simulink model "pendulum"  (R2024a)
settings: Solver=VariableStepAuto  StartTime=0.0  StopTime=10  FixedStep=0.01  MaxStep=1e-2
model workspace (MAT data in the model file):
  L = 0.2
  M = 0.054
  b = 0.01
  g = 9.81
undefined symbols (not defined in the file): X, Y, Z
libraries: sm_lib x6, nesl_utility x4
settings Model: Creator=zrway  LastModifiedBy=zrway

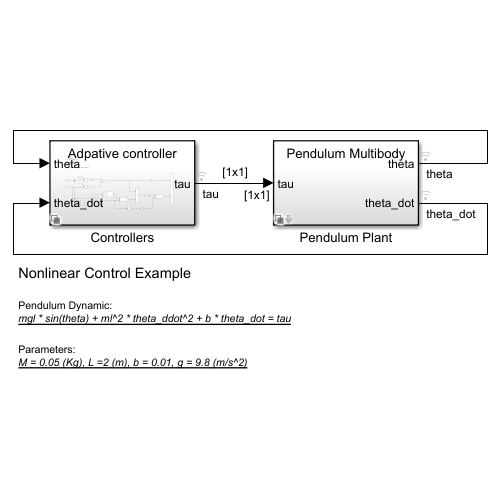
[thumbnail: Simulink's stored preview of the top-level diagram]
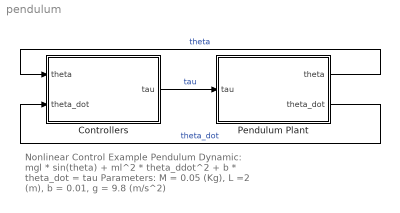
== system pendulum ==
  note: Nonlinear Control Example
      |
      | Pendulum Dynamic:
      | mgl * sin(theta) + ml^2 * theta_ddot^2 + b * theta_dot = tau
      |
      | Parameters:
      | M = 0.05 (Kg), L =2 (m), b = 0.01, g = 9.8 (m/s^2)
  Controllers : Subsystem  Variant=on  VariantControlMode=label  VariantControl=PFL controller  LabelModeActiveChoice=Adpative controller
  Pendulum Plant : Subsystem  Variant=on  VariantControlMode=label  VariantControl=Pendulum with Friction  LabelModeActiveChoice=Pendulum Multibody
  wires:
  Controllers/1(tau) -> Pendulum Plant/1(tau)  "tau"
  Pendulum Plant/1(theta) -> Controllers/1(theta)  "theta"
  Pendulum Plant/2(theta_dot) -> Controllers/2(theta_dot)  "theta_dot"

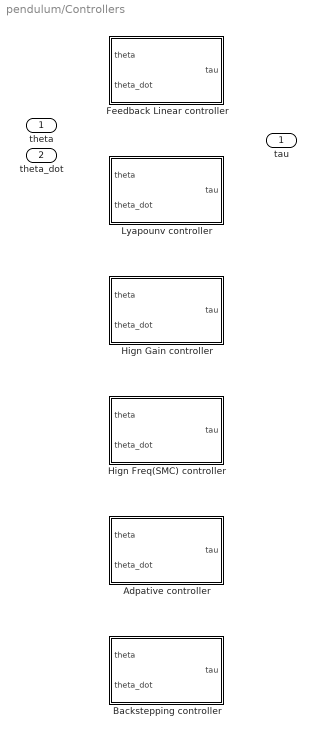
== system pendulum/Controllers ==
  theta : Inport
  theta_dot : Inport  Port=2
  Adpative controller : Subsystem  VariantControl=Adpative controller
  Backstepping controller : Subsystem  Variant=on  VariantControlMode=label  VariantControl=Backstepping controller  LabelModeActiveChoice=Backstepping controller2
  Feedback Linear controller : Subsystem  VariantControl=Feedback Linear controller
  Hign Freq(SMC) controller : Subsystem  VariantControl=Hign Freq(SMC) controller
  Hign Gain controller : Subsystem  VariantControl=Hign Gain controller
  Lyapounv controller : Subsystem  VariantControl=Lyapounv controller
  tau : Outport

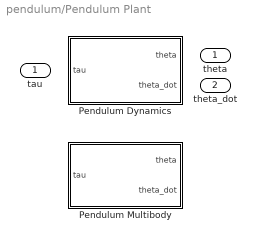
== system pendulum/Pendulum Plant ==
  tau : Inport
  Pendulum Dynamics : Subsystem  VariantControl=Pendulum Dynamics
  Pendulum Multibody : Subsystem  VariantControl=Pendulum Multibody  mask(Pendulum){L=L, W=0.01, H=0.01, m=M, rgb=[0.25 0.40 0.70], theta_init=0.4, b=b}
      mask prompts: L "Length (m)"; W "Width (m)"; H "Thickness (m)"; m "Mass (kg)"; rgb "Color [R G B]"; theta_init "Initial q (rad)"; b "Damping ratio (N*m*s/rad)"
      mask help: Pendulum simscape multibody block.
  theta : Outport
  theta_dot : Outport  Port=2

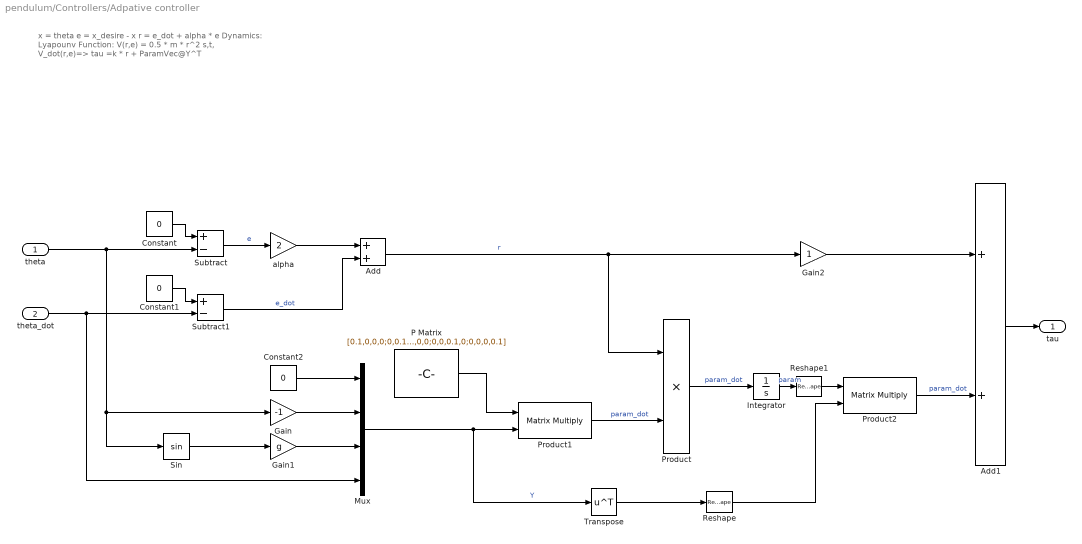
== system pendulum/Controllers/Adpative controller ==
  note: x = theta
      | e = x_desire - x
      | r = e_dot + alpha * e
      |
      | Dynamics:
      | Lyapounv Function:
      | V(r,e) = 0.5 * m * r^2
      |
      | s,t, V_dot(r,e)=> tau =k * r + ParamVec@Y^T
  theta : Inport
  theta_dot : Inport  Port=2
  Add : Sum
  Add1 : Sum
  Constant : Constant  Value=0
  Constant1 : Constant  Value=0
  Constant2 : Constant  Value=0
  Gain : Gain  Gain=-1
  Gain1 : Gain  Gain=g
  Gain2 : Gain
  Integrator : Integrator  InitialCondition=[1,0.2,1,0.1]
  Mux : Mux
  P Matrix : Constant  Value=[0.1,0,0,0;0,0.1,0,0;0,0,0.1,0;0,0,0,0.1]
  Product : Product
  Product1 : Product  Multiplication=Matrix(*)
  Product2 : Product  Multiplication=Matrix(*)
  Reshape : Reshape  OutputDimensionality=Column vector (2-D)
  Reshape1 : Reshape  OutputDimensionality=Row vector (2-D)
  Sin : Trigonometry
  Subtract : Sum  Inputs=+-
  Subtract1 : Sum  Inputs=+-
  Transpose : Math  Operator=transpose
  alpha : Gain  Gain=2
  tau : Outport
  wires:
  Subtract/1 -> alpha/1  "e"
  theta_dot/1 -> Mux/4, Subtract1/2
  theta/1 -> Sin/1, Gain/1, Subtract/2
  Add/1 -> Gain2/1, Product/1  "r"
  alpha/1 -> Add/1
  Subtract1/1 -> Add/2  "e_dot"
  Constant/1 -> Subtract/1
  Constant1/1 -> Subtract1/1
  Product/1 -> Integrator/1  "param_dot"
  Constant2/1 -> Mux/1
  Gain/1 -> Mux/2
  Gain1/1 -> Mux/3
  Sin/1 -> Gain1/1
  Mux/1 -> Transpose/1, Product1/2  "Y"
  P Matrix/1 -> Product1/1
  Product1/1 -> Product/2  "param_dot"
  Integrator/1 -> Reshape1/1  "param"
  Transpose/1 -> Reshape/1
  Product2/1 -> Add1/2  "param_dot"
  Gain2/1 -> Add1/1
  Add1/1 -> tau/1
  Reshape/1 -> Product2/2
  Reshape1/1 -> Product2/1

== system pendulum/Controllers/Backstepping controller ==
  theta : Inport
  theta_dot : Inport  Port=2
  Backstepping controller1 : Subsystem  VariantControl=Backstepping controller
  Backstepping controller2 : Subsystem  VariantControl=Backstepping controller2
  tau : Outport

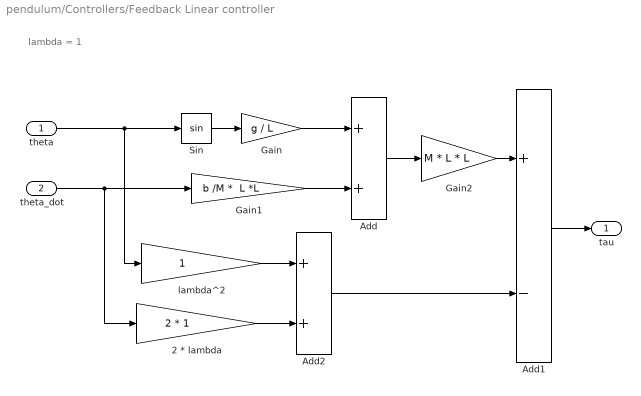
== system pendulum/Controllers/Feedback Linear controller ==
  note: lambda = 1
  theta : Inport
  theta_dot : Inport  Port=2
  2 * lambda : Gain  Gain=2 * 1
  Add : Sum
  Add1 : Sum  Inputs=+-
  Add2 : Sum
  Gain : Gain  Gain=g / L
  Gain1 : Gain  Gain="b /M *  L *L"
  Gain2 : Gain  Gain=M * L * L
  Sin : Trigonometry
  lambda^2 : Gain
  tau : Outport
  wires:
  theta/1 -> Sin/1, lambda^2/1
  Sin/1 -> Gain/1
  theta_dot/1 -> 2 * lambda/1, Gain1/1
  Gain/1 -> Add/1
  Gain1/1 -> Add/2
  Add/1 -> Gain2/1
  Gain2/1 -> Add1/1
  Add1/1 -> tau/1
  Add2/1 -> Add1/2
  2 * lambda/1 -> Add2/2
  lambda^2/1 -> Add2/1

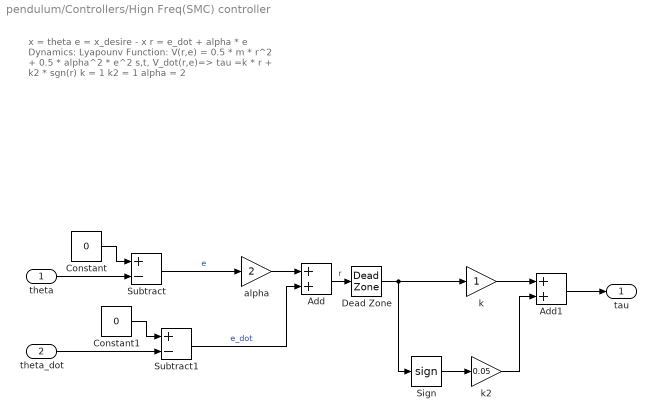
== system pendulum/Controllers/Hign Freq(SMC) controller ==
  note: x = theta
      | e = x_desire - x
      | r = e_dot + alpha * e
      |
      | Dynamics:
      | Lyapounv Function:
      | V(r,e) = 0.5 * m * r^2 + 0.5 * alpha^2 * e^2
      |
      | s,t, V_dot(r,e)=> tau =k * r + k2 * sgn(r)
      |
      | k = 1
      | k2 = 1
      | alpha = 2
  theta : Inport
  theta_dot : Inport  Port=2
  Add : Sum
  Add1 : Sum
  Constant : Constant  Value=0
  Constant1 : Constant  Value=0
  Dead Zone : DeadZone  LowerValue=-0.01  UpperValue=0.01
  Sign : Signum
  Subtract : Sum  Inputs=+-
  Subtract1 : Sum  Inputs=+-
  alpha : Gain  Gain=2
  k : Gain
  k2 : Gain  Gain=0.05
  tau : Outport
  wires:
  Constant/1 -> Subtract/1
  theta/1 -> Subtract/2
  Subtract1/1 -> Add/2  "e_dot"
  alpha/1 -> Add/1
  Subtract/1 -> alpha/1  "e"
  Add/1 -> Dead Zone/1  "r"
  theta_dot/1 -> Subtract1/2
  Constant1/1 -> Subtract1/1
  k/1 -> Add1/1
  Sign/1 -> k2/1
  k2/1 -> Add1/2
  Add1/1 -> tau/1
  Dead Zone/1 -> Sign/1, k/1

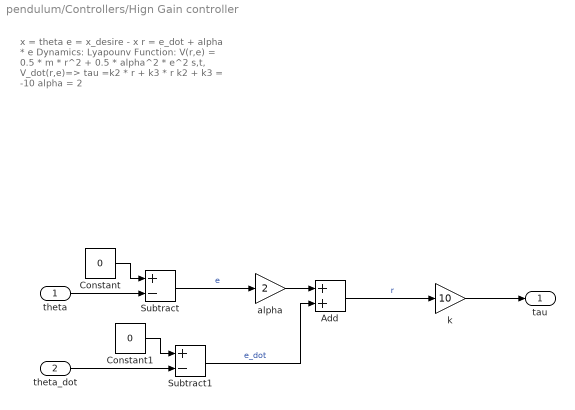
== system pendulum/Controllers/Hign Gain controller ==
  note: x = theta
      | e = x_desire - x
      | r = e_dot + alpha * e
      |
      | Dynamics:
      | Lyapounv Function:
      | V(r,e) = 0.5 * m * r^2 + 0.5 * alpha^2 * e^2
      |
      | s,t, V_dot(r,e)=> tau =k2 * r + k3 * r
      |
      | k2 + k3 = -10
      | alpha = 2
  theta : Inport
  theta_dot : Inport  Port=2
  Add : Sum
  Constant : Constant  Value=0
  Constant1 : Constant  Value=0
  Subtract : Sum  Inputs=+-
  Subtract1 : Sum  Inputs=+-
  alpha : Gain  Gain=2
  k : Gain  Gain=10
  tau : Outport
  wires:
  k/1 -> tau/1
  alpha/1 -> Add/1
  Add/1 -> k/1  "r"
  Constant/1 -> Subtract/1
  theta/1 -> Subtract/2
  Subtract/1 -> alpha/1  "e"
  Constant1/1 -> Subtract1/1
  theta_dot/1 -> Subtract1/2
  Subtract1/1 -> Add/2  "e_dot"

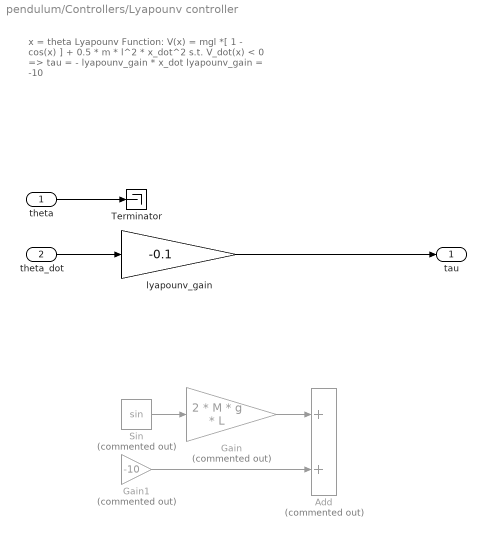
== system pendulum/Controllers/Lyapounv controller ==
  note: x = theta
      |
      | Lyapounv Function:
      | V(x) = mgl *[ 1 - cos(x) ] + 0.5 * m * l^2 * x_dot^2
      | s.t. V_dot(x) < 0
      | => tau = - lyapounv_gain * x_dot
      |
      | lyapounv_gain = -10
  theta : Inport
  theta_dot : Inport  Port=2
  Add : Sum  Commented=on
  Gain : Gain  Commented=on  Gain=2 * M * g * L
  Gain1 : Gain  Commented=on  Gain=-10
  Sin : Trigonometry  Commented=on
  Terminator : Terminator
  lyapounv_gain : Gain  Gain=-0.1
  tau : Outport
  wires:
  Sin/1 -> Gain/1
  Gain1/1 -> Add/2
  Gain/1 -> Add/1
  theta_dot/1 -> lyapounv_gain/1
  theta/1 -> Terminator/1
  lyapounv_gain/1 -> tau/1

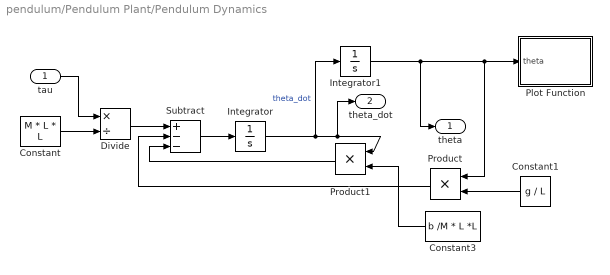
== system pendulum/Pendulum Plant/Pendulum Dynamics ==
  tau : Inport
  Constant : Constant  Value=M * L * L
  Constant1 : Constant  Value=g / L
  Constant3 : Constant  Value="b /M *  L *L"
  Divide : Product  Inputs=*/
  Integrator : Integrator
  Integrator1 : Integrator  InitialCondition=0.4  WrapState=on
  Plot Function : MATLAB Function  TreatAsAtomicUnit=on
  Product : Product
  Product1 : Product
  Subtract : Sum  Inputs=+--
  theta : Outport
  theta_dot : Outport  Port=2
  wires:
  Constant3/1 -> Product1/2
  Constant/1 -> Divide/2
  Constant1/1 -> Product/2
  tau/1 -> Divide/1
  Integrator/1 -> Product1/1, theta_dot/1, Integrator1/1  "theta_dot"
  Divide/1 -> Subtract/1
  Subtract/1 -> Integrator/1
  Product/1 -> Subtract/2
  Product1/1 -> Subtract/3
  Integrator1/1 -> Plot Function/1(theta), Product/1, theta/1

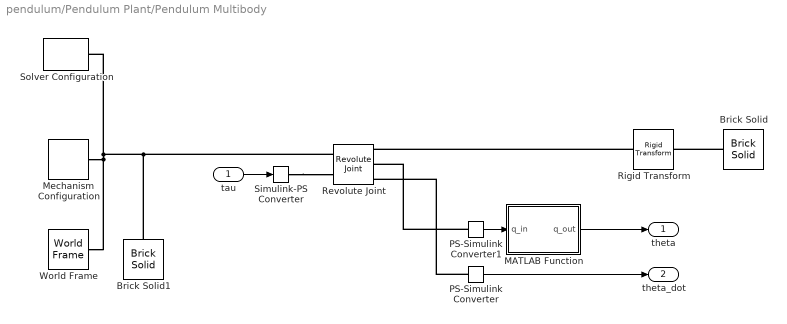
== system pendulum/Pendulum Plant/Pendulum Multibody ==
  tau : Inport
  Brick Solid : sm_lib/Body Elements/Brick Solid  BrickDimensions=[L H W]  BrickDimensionsUnits=m  ExportEntireGeometry=off  InertiaType=CalculateFromGeometry  BasedOnType=Mass  Density=rho  DensityUnits=kg/m^3  Mass=m  MassUnits=kg  CenterOfMass=[0 0 0]  CenterOfMassUnits=m  MomentsOfInertia=[1 1 1]  MomentsOfInertiaUnits=kg*m^2  ProductsOfInertia=[0 0 0]  ProductsOfInertiaUnits=kg*m^2  GraphicType=FromGeometry  MarkerShape=Sphere  MarkerSize=10  GraphicVisPropType=SimpleVisualProperties  GraphicDiffuseColor=rgb  GraphicOpacity=1  GraphicSpecularColor=[0.5 0.5 0.5 1.0]  GraphicAmbientColor=[0.15 0.15 0.15 1.0]  GraphicEmissiveColor=[0.0 0.0 0.0 1.0]  GraphicShininess=75  DoExposeReferenceFrame=on  SerializedFrames=<Frames/>
  Brick Solid1 : sm_lib/Body Elements/Brick Solid  BrickDimensions=[0.04 0.04 0.04]  BrickDimensionsUnits=m  ExportEntireGeometry=off  InertiaType=CalculateFromGeometry  BasedOnType=Density  Density=1000  DensityUnits=kg/m^3  Mass=1  MassUnits=kg  CenterOfMass=[0 0 0]  CenterOfMassUnits=m  MomentsOfInertia=[1 1 1]  MomentsOfInertiaUnits=kg*m^2  ProductsOfInertia=[0 0 0]  ProductsOfInertiaUnits=kg*m^2  GraphicType=FromGeometry  MarkerShape=Sphere  MarkerSize=10  GraphicVisPropType=SimpleVisualProperties  GraphicDiffuseColor=[0.80 0.45 0]  GraphicOpacity=1  GraphicSpecularColor=[0.5 0.5 0.5 1.0]  GraphicAmbientColor=[0.15 0.15 0.15 1.0]  GraphicEmissiveColor=[0.0 0.0 0.0 1.0]  GraphicShininess=75  DoExposeReferenceFrame=on  SerializedFrames=<Frames/>
  MATLAB Function : MATLAB Function  TreatAsAtomicUnit=on
  Mechanism Configuration : sm_lib/Utilities/Mechanism Configuration  UniformGravity=Constant  GravityVector=[0 -9.80665 0]  GravityVectorUnits=m/s^2  LinearizationDelta=0.001  JointModeTransitionNonlinearIterations=2
  PS-Simulink Converter : nesl_utility/PS-Simulink Converter  PhysicalDomain=network_engine_domain  SubClassName=ps_output  LeftPortType=input  RightPortType=output  PseudoPeriodic=off  Frequencies=[]  VectorFormat=1-D array  Unit=rad/s  AffineConversion=off
  PS-Simulink Converter1 : nesl_utility/PS-Simulink Converter  PhysicalDomain=network_engine_domain  SubClassName=ps_output  LeftPortType=input  RightPortType=output  PseudoPeriodic=off  Frequencies=[]  VectorFormat=inherit  Unit=rad  AffineConversion=off
  Revolute Joint : sm_lib/Joints/Revolute Joint  JointMode=Normal  CompositeWrenchDir=FollowerOnBase  CompositeWrenchFrame=BaseFrame  SenseConstraintForce=off  SenseConstraintTorque=off  SenseTotalForce=off  SenseTotalTorque=off  PositionTargetSpecify=on  PositionTargetPriority=High  PositionTargetValue=-pi / 2 + theta_init  PositionTargetValueUnits=rad  VelocityTargetSpecify=on  VelocityTargetPriority=Low  VelocityTargetValue=0.0001  VelocityTargetValueUnits=rad/s  EquilibriumPosition=pi / 2  EquilibriumPositionUnits=rad  SpringStiffness=0  SpringStiffnessUnits=N*m/deg  DampingCoefficient=b  DampingCoefficientUnits=N*m*s/rad  LowerLimitSpecify=off  LowerLimitBound=-90  LowerLimitBoundUnits=deg  LowerLimitStiffness=1e4  LowerLimitStiffnessUnits=N*m/deg  LowerLimitDamping=10  LowerLimitDampingUnits=N*m/(deg/s)  LowerLimitTransitionRegionWidth=0.1  LowerLimitTransitionRegionWidthUnits=deg  UpperLimitSpecify=off  UpperLimitBound=90  UpperLimitBoundUnits=deg  UpperLimitStiffness=1e4  UpperLimitStiffnessUnits=N*m/deg  UpperLimitDamping=10  UpperLimitDampingUnits=N*m/(deg/s)  UpperLimitTransitionRegionWidth=0.1  UpperLimitTransitionRegionWidthUnits=deg  TorqueActuationMode=InputTorque  MotionActuationMode=ComputedMotion  SensePosition=on  SenseVelocity=on  SenseAcceleration=off  SenseTorqueForce=off  SenseLowerLimitTorqueForce=off  SenseUpperLimitTorqueForce=off
  Rigid Transform : sm_lib/Frames and Transforms/Rigid Transform  RotationMethod=None  FollAlignAxisA=+X  BaseAlignAxisA=+Y  FollAlignAxisB=+Y  BaseAlignAxisB=+Z  RotationStandardAxis=+Z  RotationAngle=0  RotationAngleUnits=deg  RotationArbitraryAxis=[0 0 1]  RotationSequenceAxes=FollowerAxes  RotationSequence=XYX  RotationSequenceAngles=[0 0 0]  RotationSequenceAnglesUnits=deg  RotationMatrix=[1 0 0;0 1 0;0 0 1]  Quaternion=[1 0 0 0]  TranslationMethod=StandardAxis  TranslationCartesianOffset=[0 0 0]  TranslationCartesianOffsetUnits=m  TranslationStandardAxis=-X  TranslationStandardOffset=L / 2  TranslationStandardOffsetUnits=m  TranslationROffset=0  TranslationROffsetUnits=m  TranslationThetaOffset=0  TranslationThetaOffsetUnits=deg  TranslationZOffset=0  TranslationZOffsetUnits=m
  Simulink-PS Converter : nesl_utility/Simulink-PS Converter  PhysicalDomain=network_engine_domain  SubClassName=ps_input  LeftPortType=input  RightPortType=output  PseudoPeriodic=off  Frequencies=[]  NoiseDistribution=none  NoiseParameters=[]  Unit=N*m  AffineConversion=off  FilteringAndDerivatives=provide  SimscapeFilterOrder=1  InputFilterTimeConstant=0.001  UdotUserProvided=0
  Solver Configuration : nesl_utility/Solver Configuration  PhysicalDomain=network_engine_domain  SubClassName=solver  LeftPortType=input  RightPortType=generic  Tones=[]  Harmonics=[]  SimulateNoise=off  Profile=off  UseLocalSampling=off  EnableSwitchedLinearOptims=on  FrequencyDomain=off  UseCCode=off  RelTol=0.001  AbsTol=0.001  MinStep=1e-09  ToWorkspace=off  RevertToSquareIcSolve=off  NumHomotopyIterations=100  PhasorMode=off  PhasorModeNumHarmonics=1  ConsistencySolver=NEWTON_XTOL_AFTER_FTOL  IndexReductionMethod=DerivativeReplacement  DoDC=off  ResidualTolerance=1e-09  ConsistencyTolSource=GLOBAL  ConsistencyAbsTol=0.001  ConsistencyRelTol=0.001  ConsistencyTolFactor=0.001  UseLocalSolver=off  LocalSolverChoice=NE_BACKWARD_EULER_ADVANCER  ResolveIndetEquations=on  FunctionEvalNumThread=1  LocalSolverSampleTime=0.001  DoFixedCost=off  MaxNonlinIter=3  MaxModeIter=2  ComputeImpulses=off  ImpulseIterations=2  LinearAlgebra=auto  LinearAlgebraNumThread=0  EquationFormulation=NE_TIME_EF  DelaysMemoryBudget=1024  AutomaticFiltering=on  FilteringTimeConstant=0.001  PartitionStorageMethod=AS_NEEDED  PartitionMemoryBudget=1024  PartitionMethod=ROBUST  MultibodyUseLocalSolver=off  MultibodyLocalSolverChoice=ODE1  MultibodyLocalSolverSampleTime=0.001
  World Frame : sm_lib/Frames and Transforms/World Frame
  theta : Outport
  theta_dot : Outport  Port=2
  wires:
  PS-Simulink Converter1/1 -> MATLAB Function/1(q_in)
  tau/1 -> Simulink-PS Converter/1
  MATLAB Function/1(q_out) -> theta/1
  PS-Simulink Converter/1 -> theta_dot/1
  connections:
  Brick Solid1/RConn1 -- World Frame/RConn1 -- Mechanism Configuration/RConn1 -- Solver Configuration/RConn1 -- Revolute Joint/LConn1
  PS-Simulink Converter/LConn1 -- Revolute Joint/RConn3
  Brick Solid/RConn1 -- Rigid Transform/RConn1
  PS-Simulink Converter1/LConn1 -- Revolute Joint/RConn2
  Simulink-PS Converter/RConn1 -- Revolute Joint/LConn2
  Rigid Transform/LConn1 -- Revolute Joint/RConn1

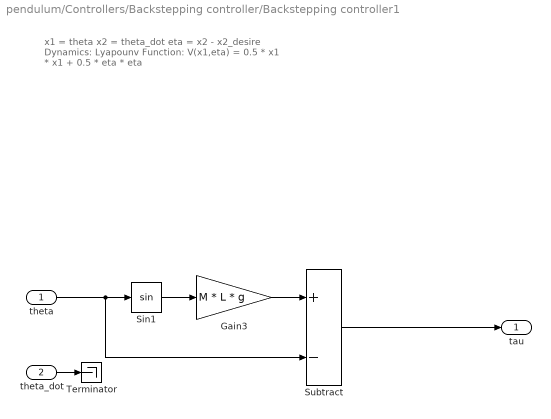
== system pendulum/Controllers/Backstepping controller/Backstepping controller1 ==
  note: x1 = theta
      | x2 = theta_dot
      |
      | eta = x2 - x2_desire
      |
      | Dynamics:
      | Lyapounv Function:
      | V(x1,eta) = 0.5 * x1 * x1 + 0.5 * eta * eta
  theta : Inport
  theta_dot : Inport  Port=2
  Gain3 : Gain  Gain=M * L * g
  Sin1 : Trigonometry
  Subtract : Sum  Inputs=+-
  Terminator : Terminator
  tau : Outport
  wires:
  Sin1/1 -> Gain3/1
  theta/1 -> Subtract/2, Sin1/1
  Gain3/1 -> Subtract/1
  theta_dot/1 -> Terminator/1
  Subtract/1 -> tau/1

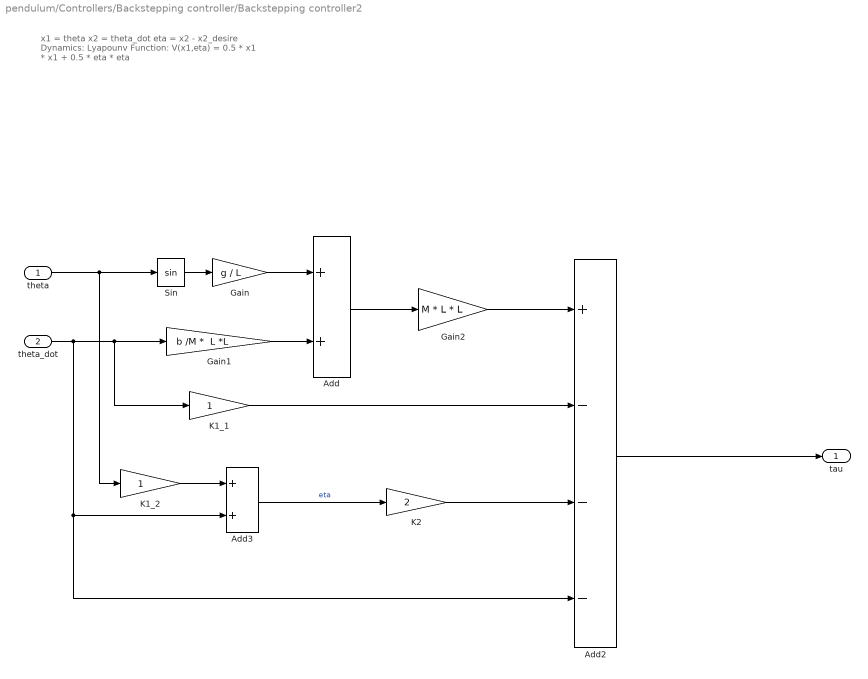
== system pendulum/Controllers/Backstepping controller/Backstepping controller2 ==
  note: x1 = theta
      | x2 = theta_dot
      |
      | eta = x2 - x2_desire
      |
      | Dynamics:
      | Lyapounv Function:
      | V(x1,eta) = 0.5 * x1 * x1 + 0.5 * eta * eta
  theta : Inport
  theta_dot : Inport  Port=2
  Add : Sum
  Add2 : Sum  Inputs=+---
  Add3 : Sum
  Gain : Gain  Gain=g / L
  Gain1 : Gain  Gain="b /M *  L *L"
  Gain2 : Gain  Gain=M * L * L
  K1_1 : Gain
  K1_2 : Gain
  K2 : Gain  Gain=2
  Sin : Trigonometry
  tau : Outport
  wires:
  K1_2/1 -> Add3/1
  K2/1 -> Add2/3
  Sin/1 -> Gain/1
  Add3/1 -> K2/1  "eta"
  Add/1 -> Gain2/1
  Gain1/1 -> Add/2
  Gain2/1 -> Add2/1
  K1_1/1 -> Add2/2
  Gain/1 -> Add/1
  theta_dot/1 -> Add3/2, Add2/4, K1_1/1, Gain1/1
  theta/1 -> K1_2/1, Sin/1
  Add2/1 -> tau/1

== matlab function pendulum/Pendulum Plant/Pendulum Multibody/MATLAB Function ==
  data: q_in input; q_out output
function q_out = fcn(q_in)

q_out = q_in + pi / 2;

== matlab function pendulum/Pendulum Plant/Pendulum Dynamics/Plot Function ==
  data: theta input
function  fcn(theta)

% pendulum plot
% dynamics:
%    
figure(999);
cla(gca);

x = 1 * cos(theta + pi / 2);
y = 1 * sin(theta + pi / 2);
plot([0,x],[0,y],"LineWidth",1.5,"Color","g")
xlim([-2,2])
ylim([-1,2])
hold on
scatter(0,0,80,"b","square","filled")
scatter(x,y,100,"r", "o", "filled")
